simulink model "recordTEST"  (R2019a)
settings: Solver=FixedStepAuto  StartTime=0.0  StopTime=inf  RelTol=1e-3  EnableMultiTasking=on
undefined symbols (not defined in the file or in its folder): daq, fdesignblkfcn, gcbh
libraries: dspfdesign x10, daqlib x2, dsparch4 x1, dspstat3 x1
settings Model: ExtModeTrigDuration=2  Creator=Kusunoki  LastModifiedBy=Owner
settings OptimizationCC: EnhancedBackFolding=on  PassReuseOutputArgsAs=Individual arguments  MaxStackSize=64  OptimizeBlockOrder=speed  DifferentSizesBufferReuse=on  OptimizationCustomize=off
settings DebuggingCC: ParameterTunabilityLossMsg=error
settings HardwareCC: ProdBitPerInt=16  ProdBitPerPointer=16  ProdBitPerSizeT=16  ProdBitPerPtrDiffT=16  ProdLargestAtomicFloat=None  ProdWordSize=8  ProdHWDeviceType=Atmel->AVR
settings SFSimCC: MATLABDynamicMemAlloc=off
settings RTWCC: SystemTargetFile=ert.tlc  HardwareBoard=Arduino Mega 2560  TLCOptions=-aInlineSetEventsForThisBaseRateFcn=TLC_FALSE -aSuppressMultiTaskScheduler=TLC_FALSE -aRateBasedStepFcn=1  TemplateMakefile=ert_default_tmf  GenerateReport=on  Toolchain=Arduino AVR  BuildConfiguration=Faster Runs  IncludeHyperlinkInReport=on  LaunchReport=on  GenerateTraceInfo=on  GenerateTraceReport=on  GenerateTraceReportSl=on  GenerateTraceReportSf=on  GenerateTraceReportEml=on
settings CodeAppCC: ForceParamTrailComments=on  IgnoreCustomStorageClasses=off  OperatorAnnotations=on  SimulinkDataObjDesc=on  SFDataObjDesc=on  InsertBlockDesc=on
settings ERTTargetCC: SupportContinuousTime=on  SupportVariableSizeSignals=on  ExtModeStaticAllocSize=2048

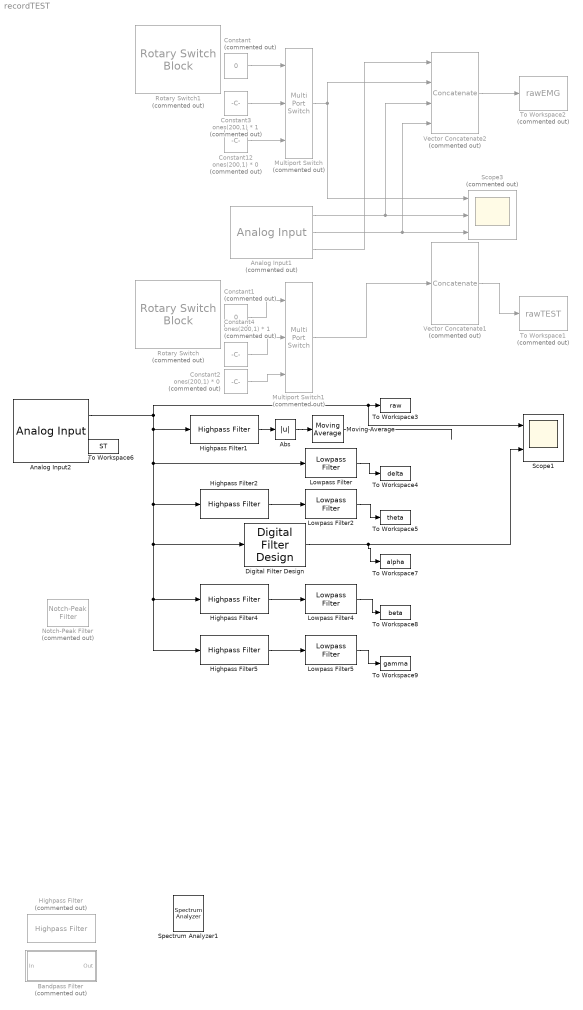
== system recordTEST ==
  Abs : Abs
  Analog Input1 : daqlib/Analog Input  Commented=on  DeviceMenu=ni Dev1 (USB-6000)  Device=ni Dev1 (USB-6000)  ObjConstructor=daq.createSession('ni')  NChannelsSelected=2  Channels=1$ai0$$Dev1$1$1$1$1$#1$ai1$$Dev1$1$1$1$1$#0$ai2$$Dev1$1$1$1$1$#0$ai3$$Dev1$1$1$1$1$#0$ai4$$Dev1$1$1$1$1$#0$ai5$$Dev1$1$1$1$1$#0$ai6$$Dev1$1$1$1$1$#0$ai7$$Dev1$1$1$1$1$#  NPorts=1 per channel  SampleRate=2000  ActualRate=2000  ScansPerTrigger=200  OutputTimestamp=on  AcqMode=0  NumFrameBuffer=100  OutputTriggertime=off
      settings: SourceProductName=Data Acquisition Toolbox  SourceProductBaseCode=DA
  Analog Input2 : daqlib/Analog Input  DeviceMenu=ni Dev1 (USB-6000)  Device=ni Dev1 (USB-6000)  ObjConstructor=daq.createSession('ni')  NChannelsSelected=3  Channels=1$ai0$$Dev1$1$1$1$1$#1$ai1$$Dev1$1$1$1$1$#1$ai2$$Dev1$1$1$1$1$#0$ai3$$Dev1$1$1$1$1$#0$ai4$$Dev1$1$1$1$1$#0$ai5$$Dev1$1$1$1$1$#0$ai6$$Dev1$1$1$1$1$#0$ai7$$Dev1$1$1$1$1$#  NPorts=1 for all channels  SampleRate=1000  ActualRate=1000.2501  ScansPerTrigger=200  OutputTimestamp=on  AcqMode=0  NumFrameBuffer=100  OutputTriggertime=off
      settings: SourceProductName=Data Acquisition Toolbox  SourceProductBaseCode=DA
  Bandpass Filter : Subsystem  Commented=on  DialogController=fdesignblkfcn  InitFcn=fdesignblkfcn(gcbh, {'InitFcn'});  mask(Bandpass Filter){}
      mask help: Design a bandpass filter
      settings: CopyFcn=fdesignblkfcn(gcbh, {'CopyFcn'});
      mask Help: helpview(mapfilelocation('dsp'), 'dspbandpassfilter');
      mask Display: disp('Bandpass');
  Constant : Constant  Commented=on  Value=0
  Constant1 : Constant  Commented=on  Value=0
  Constant12 : Constant  Commented=on  Value=ones(200,1) * 0
  Constant2 : Constant  Commented=on  Value=ones(200,1) * 0
  Constant3 : Constant  Commented=on  Value=ones(200,1) * 1
  Constant4 : Constant  Commented=on  Value=ones(200,1) * 1
  Digital Filter Design : dsparch4/Digital Filter Design  mwdsp_browser_bugfix_var=off
  Highpass Filter : dspfdesign/Highpass Filter  Commented=on  FilterType=FIR  DesignForMinimumOrder=on  FilterOrder=50  StopbandFrequency=0.1  PassbandFrequency=0.2  StopbandAttenuation=80  PassbandRipple=0.1  InheritSampleRate=off  SampleRate=2000  SimulateUsing=Interpreted execution  roundingMode=Floor  coeffsDataTypeStr=fixdt(1,16)
      settings: SourceProductName=DSP System Toolbox
  Highpass Filter1 : dspfdesign/Highpass Filter  FilterType=IIR  DesignForMinimumOrder=on  FilterOrder=50  StopbandFrequency=3  PassbandFrequency=4  StopbandAttenuation=80  PassbandRipple=0.1  InheritSampleRate=on  SampleRate=2000  SimulateUsing=Interpreted execution  roundingMode=Floor  coeffsDataTypeStr=fixdt(1,16)
      settings: SourceProductName=DSP System Toolbox
  Highpass Filter2 : dspfdesign/Highpass Filter  FilterType=IIR  DesignForMinimumOrder=on  FilterOrder=50  StopbandFrequency=3  PassbandFrequency=4  StopbandAttenuation=80  PassbandRipple=0.1  InheritSampleRate=on  SampleRate=2000  SimulateUsing=Interpreted execution  roundingMode=Floor  coeffsDataTypeStr=fixdt(1,16)
      settings: SourceProductName=DSP System Toolbox
  Highpass Filter4 : dspfdesign/Highpass Filter  FilterType=IIR  DesignForMinimumOrder=on  FilterOrder=50  StopbandFrequency=13  PassbandFrequency=14  StopbandAttenuation=80  PassbandRipple=0.1  InheritSampleRate=on  SampleRate=2000  SimulateUsing=Interpreted execution  roundingMode=Floor  coeffsDataTypeStr=fixdt(1,16)
      settings: SourceProductName=DSP System Toolbox
  Highpass Filter5 : dspfdesign/Highpass Filter  FilterType=IIR  DesignForMinimumOrder=on  FilterOrder=50  StopbandFrequency=34  PassbandFrequency=35  StopbandAttenuation=80  PassbandRipple=0.1  InheritSampleRate=on  SampleRate=2000  SimulateUsing=Interpreted execution  roundingMode=Floor  coeffsDataTypeStr=fixdt(1,16)
      settings: SourceProductName=DSP System Toolbox
  Lowpass Filter : dspfdesign/Lowpass Filter  FilterType=IIR  DesignForMinimumOrder=on  FilterOrder=50  PassbandFrequency=3  StopbandFrequency=4  PassbandRipple=0.1  StopbandAttenuation=80  InheritSampleRate=on  SampleRate=2000  SimulateUsing=Interpreted execution  roundingMode=Floor  coeffsDataTypeStr=fixdt(1,16)
  Lowpass Filter2 : dspfdesign/Lowpass Filter  FilterType=IIR  DesignForMinimumOrder=on  FilterOrder=50  PassbandFrequency=7  StopbandFrequency=8  PassbandRipple=0.1  StopbandAttenuation=80  InheritSampleRate=on  SampleRate=2000  SimulateUsing=Interpreted execution  roundingMode=Floor  coeffsDataTypeStr=fixdt(1,16)
  Lowpass Filter4 : dspfdesign/Lowpass Filter  FilterType=IIR  DesignForMinimumOrder=on  FilterOrder=50  PassbandFrequency=35  StopbandFrequency=36  PassbandRipple=0.1  StopbandAttenuation=80  InheritSampleRate=on  SampleRate=2000  SimulateUsing=Interpreted execution  roundingMode=Floor  coeffsDataTypeStr=fixdt(1,16)
  Lowpass Filter5 : dspfdesign/Lowpass Filter  FilterType=IIR  DesignForMinimumOrder=on  FilterOrder=50  PassbandFrequency=55  StopbandFrequency=56  PassbandRipple=0.1  StopbandAttenuation=80  InheritSampleRate=on  SampleRate=2000  SimulateUsing=Interpreted execution  roundingMode=Floor  coeffsDataTypeStr=fixdt(1,16)
  Moving Average : dspstat3/Moving Average  Method=Sliding window  ForgettingFactorPort=off  SpecifyWindowLength=on  WindowLength=200  ForgettingFactor=0.9  SimulateUsing=Code generation
  Multiport Switch : MultiPortSwitch  Commented=on  DataPortOrder=Specify indices  DataPortIndices={1,0}
  Multiport Switch1 : MultiPortSwitch  Commented=on  DataPortOrder=Specify indices  DataPortIndices={1,0}
  Notch-Peak Filter : dspfdesign/Notch-Peak Filter  Commented=on  Specification=Bandwidth and center frequency  BandwidthPort=off  Bandwidth=2  QualityFactorPort=off  QualityFactor=5  CenterFrequencyPort=off  CenterFrequency=60  BandwidthCoefficientPort=off  BandwidthCoefficient=0.72654  CenterFrequencyCoefficientPort=off  CenterFrequencyCoefficient=0  Output=Notch and Peak  InheritSampleRate=off  SampleRate=2000  SimulateUsing=Code generation
      settings: SourceProductName=DSP System Toolbox  SourceProductBaseCode=DS
  Rotary Switch : RotarySwitchBlock  Commented=on
      settings: Values={{'0：relax', '1 : grip'}, [0 1]}
  Rotary Switch1 : RotarySwitchBlock  Commented=on
      settings: Values={{'0 : relax', '1 : grip'}, [0 1]}
  Scope1 : Scope  NumInputPorts=2
  Scope3 : Scope  Commented=on  NumInputPorts=3
  Spectrum Analyzer1 : SpectrumAnalyzer  NumInputPorts=2
  To Workspace1 : ToWorkspace  Commented=on  VariableName=rawTEST  SampleTime=-1
      settings: Save2DSignal=2-D array (concatenate along first dimension)
  To Workspace2 : ToWorkspace  Commented=on  VariableName=rawEMG  SampleTime=-1
      settings: Save2DSignal=2-D array (concatenate along first dimension)
  To Workspace3 : ToWorkspace  VariableName=raw  SampleTime=-1
      settings: Save2DSignal=2-D array (concatenate along first dimension)
  To Workspace4 : ToWorkspace  VariableName=delta  SampleTime=-1
      settings: Save2DSignal=2-D array (concatenate along first dimension)
  To Workspace5 : ToWorkspace  VariableName=theta  SampleTime=-1
      settings: Save2DSignal=2-D array (concatenate along first dimension)
  To Workspace6 : ToWorkspace  VariableName=ST  SampleTime=-1
      settings: Save2DSignal=2-D array (concatenate along first dimension)
  To Workspace7 : ToWorkspace  VariableName=alpha  SampleTime=-1
      settings: Save2DSignal=2-D array (concatenate along first dimension)
  To Workspace8 : ToWorkspace  VariableName=beta  SampleTime=-1
      settings: Save2DSignal=2-D array (concatenate along first dimension)
  To Workspace9 : ToWorkspace  VariableName=gamma  SampleTime=-1
      settings: Save2DSignal=2-D array (concatenate along first dimension)
  Vector Concatenate1 : Concatenate  Commented=on  NumInputs=3  Mode=Multidimensional array  ConcatenateDimension=2
  Vector Concatenate2 : Concatenate  Commented=on  NumInputs=4  Mode=Multidimensional array  ConcatenateDimension=2
  wires:
  Constant12/1 -> Multiport Switch/3
  Multiport Switch/1 -> Vector Concatenate2/2, Scope3/1
  Constant3/1 -> Multiport Switch/2
  Constant/1 -> Multiport Switch/1
  Analog Input1/1 -> Scope3/2, Vector Concatenate2/3
  Analog Input1/2 -> Vector Concatenate2/4, Scope3/3
  Vector Concatenate2/1 -> To Workspace2/1
  Analog Input1/3 -> Vector Concatenate2/1
  Vector Concatenate1/1 -> To Workspace1/1
  Multiport Switch1/1 -> Vector Concatenate1/2
  Constant4/1 -> Multiport Switch1/2
  Constant1/1 -> Multiport Switch1/1
  Constant2/1 -> Multiport Switch1/3
  Analog Input2/2 -> To Workspace6/1
  Analog Input2/1 -> Highpass Filter1/1, Highpass Filter2/1, Highpass Filter4/1, Highpass Filter5/1, Digital Filter Design/1, Lowpass Filter/1, Scope1/1, To Workspace3/1
  Highpass Filter4/1 -> Lowpass Filter4/1
  Highpass Filter5/1 -> Lowpass Filter5/1
  Highpass Filter2/1 -> Lowpass Filter2/1
  Lowpass Filter/1 -> To Workspace4/1
  Digital Filter Design/1 -> To Workspace7/1, Scope1/2
  Lowpass Filter5/1 -> To Workspace9/1
  Lowpass Filter4/1 -> To Workspace8/1
  Lowpass Filter2/1 -> To Workspace5/1
  Highpass Filter1/1 -> Abs/1
  Abs/1 -> Moving Average/1
  Moving Average/1 -> ?

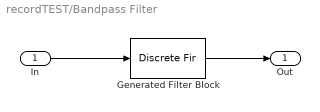
== system recordTEST/Bandpass Filter ==
  In : Inport
  Generated Filter Block : DiscreteFir  Tag=BlockMethodSubSystem  Coefficients=[-0.0008992291487744296 0.0016414518747943749 0.0031352071842225397 -0.0040707550828814922 -0.0063731852227904111 0.0074874286806090491 0.0098354319566295711 -0.010189316513446216 -0.011302794465874122 0.0096929185841818435 0.0079428653987464216 -0.0031368247881221642 0.0028299878877943137 -0.011508674243001471 -0.022080136219461581 0.034245325424507672 0.048356661648905473 -0.062355369169884239 -0.077503478162593897 0.090687768153125653 0.10353171105844157 -0.11297860084229834 -0.12035866024978455 0.12379360801539134 0.12379360801539134 -0.12035866024978455 -0.11297860084229834 0.10353171105844157 0.090687768153125653 -0.077503478162593897 -0.062355369169884239 0.048356661648905473 0.034245325424507672 -0.022080136219461581 -0.011508674243001471 0.0028299878877943137 -0.0031368247881221642 0.0079428653987464216 0.0096929185841818435 -0.011302794465874122 -0.010189316513446216 0.0098354319566295711 0.0074874286806090491 -0.0063731852227904111 -0.0040707550828814922 0.0031352071842225397 0.0016414518747943749 -0.0008992291487744296]  InputProcessing=Columns as channels (frame based)
  Out : Outport
  wires:
  In/1 -> Generated Filter Block/1
  Generated Filter Block/1 -> Out/1
